simulink model "ES005A_TmplMonr"  (R2013b)
settings: Solver=ode45  StartTime=0.0  StopTime=2  RelTol=1e-3
values from neighbouring files (symbols this model uses):
  ELECGLBPRM_STRTUPSTTMPLMONININTESTSTRT_CNT_U08 = DataDict.Constant    [ES005A_TmplMonr_DataDict.m]
  IninFlt = DataDict.NTC    [ES005A_TmplMonr_DataDict.m]
  RtFlt = DataDict.NTC    [ES005A_TmplMonr_DataDict.m]
  SpiConf_SpiChannel_TmplMonrCh1 = DataDict.Constant    [ES005A_TmplMonr_DataDict.m]
  SpiConf_SpiChannel_TmplMonrCh2 = DataDict.Constant    [ES005A_TmplMonr_DataDict.m]
  SpiConf_SpiChannel_TmplMonrCh3 = DataDict.Constant    [ES005A_TmplMonr_DataDict.m]
  SpiConf_SpiSequence_TmplMonrSeq1 = DataDict.Constant    [ES005A_TmplMonr_DataDict.m]
  SpiConf_SpiSequence_TmplMonrSeq2 = DataDict.Constant    [ES005A_TmplMonr_DataDict.m]
  SpiConf_SpiSequence_TmplMonrSeq3 = DataDict.Constant    [ES005A_TmplMonr_DataDict.m]
  STD_HIGH = DataDict.Constant    [ES005A_TmplMonr_DataDict.m]
  STD_LOW = DataDict.Constant    [ES005A_TmplMonr_DataDict.m]
  TMPLMONRCFGREG1READVAL_CNT_U16 = DataDict.Constant    [ES005A_TmplMonr_DataDict.m]
  TMPLMONRCFGREG1WRVAL_CNT_U16 = DataDict.Constant    [ES005A_TmplMonr_DataDict.m]
  TMPLMONRSTSREG2READVAL_CNT_U16 = DataDict.Constant    [ES005A_TmplMonr_DataDict.m]
  TMPLMONRWDGMODKEYWORD1_CNT_U16 = DataDict.Constant    [ES005A_TmplMonr_DataDict.m]
  TMPLMONRWDGMODKEYWORD2_CNT_U16 = DataDict.Constant    [ES005A_TmplMonr_DataDict.m]
  TMPLMONRWDGMODKEYWORD3_CNT_U16 = DataDict.Constant    [ES005A_TmplMonr_DataDict.m]
undefined symbols (not defined in the file or in its folder): TrigReg1
libraries: simulink x12
(part 2 of 4)

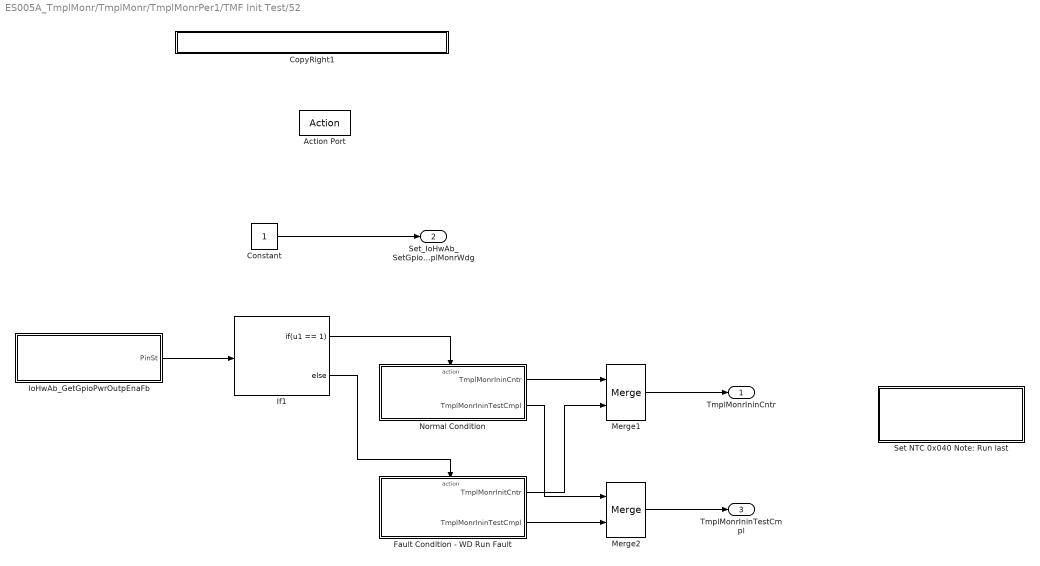
== system ES005A_TmplMonr/TmplMonr/TmplMonrPer1/TMF Init Test/52 ==
  Action Port : ActionPort  ActionType=case
  Constant : Constant  OutDataTypeStr=boolean
  CopyRight1 : Subsystem  Description=|  mask(Copyright Information){none=on}
      | Copyright info block.                                               
      |                                                                     
      | Place copyright information at the top of every subsystem in design.
      mask prompts: none "No parameters"
      mask help: Place copyright information at the top of every subsystem in design.
      mask Display:
      | NxtrConf = 'Nexteer Confidential';
      | 
      | sys = bdroot; %handle for the current model ("system")
      | first = get_param(sys,'Created');
      | first = first(end-3:end);  %year is last four digits
      | 
      | last = get_param(sys,'LastModifiedDate');
      | if isempty(last)
      |     last = datestr(now,'yyyy');
      | else
      |     last = last(end-3:end);
      | end
      | 
      | if strcmp(first,last)
      |     fprintf('%s -- Copyright %s Nexteer',NxtrConf,first)
      | else
      |     fprintf('%s -- %s%s- %s Nexteer',NxtrConf,char(169),first,last)
      | end
  Fault Condition - WD Run Fault : Subsystem  RequirementInfo={} %GIDa_b93698f8_2763_40bb_9d1b_225acd7973d3
  If1 : If  IfExpression=u1 == 1
  IoHwAb_GetGpioPwrOutpEnaFb : Subsystem
  Merge1 : Merge
  Merge2 : Merge
  Normal Condition : Subsystem  RequirementInfo={'linktype_rmi_doors' '0000c46a (/ESG Group/FDD Module Requirements/EA4 Specific/ES005A_TmplMonr)' '#ES005A_164' 'true' 'REQ: ES005A_164' '' } %GIDa_785a744b_ba8b_461e_b98b_5c61c0bc0772
  Set NTC 0x040 Note: Run last : Subsystem  RequirementInfo="{'linktype_rmi_doors' '0000c46a (/ESG Group/FDD Module Requirements/EA4 Specific/ES005A_TmplMonr)' '#ES005A_183' 'true' 'REQ:  ES005A_183' '' } %GIDa_d81dec6a_41a1_4ea0_a985_1fcdbb0d2b96"
  TmplMonrIninCntr : Outport
  Set_IoHwAb_SetGpioTmplMonrWdg : Outport  Port=2
  TmplMonrIninTestCmpl : Outport  Port=3
  wires:
  If1/1 -> Normal Condition/Action
  If1/2 -> Fault Condition - WD Run Fault/Action
  IoHwAb_GetGpioPwrOutpEnaFb/1(PinSt) -> If1/1
  Normal Condition/1(TmplMonrIninCntr) -> Merge1/1
  Fault Condition - WD Run Fault/1(TmplMonrInitCntr) -> Merge1/2
  Constant/1 -> Set_IoHwAb_SetGpioTmplMonrWdg/1
  Merge1/1 -> TmplMonrIninCntr/1
  Merge2/1 -> TmplMonrIninTestCmpl/1
  Normal Condition/2(TmplMonrIninTestCmpl) -> Merge2/1
  Fault Condition - WD Run Fault/2(TmplMonrIninTestCmpl) -> Merge2/2

== system ES005A_TmplMonr/TmplMonr/TmplMonrPer1/TMF Init Test/9-10, 14-16 ==
  Action Port : ActionPort  ActionType=case
  Constant : Constant  Value=0  OutDataTypeStr=boolean
  Constant2 : Constant  OutDataTypeStr=uint8
  Constant3 : Constant  Value=STD_HIGH  OutDataTypeStr=boolean
  CopyRight1 : Subsystem  Description=|  mask(Copyright Information){none=on}
      | Copyright info block.                                               
      |                                                                     
      | Place copyright information at the top of every subsystem in design.
      mask prompts: none "No parameters"
      mask help: Place copyright information at the top of every subsystem in design.
      mask Display:
      | NxtrConf = 'Nexteer Confidential';
      | 
      | sys = bdroot; %handle for the current model ("system")
      | first = get_param(sys,'Created');
      | first = first(end-3:end);  %year is last four digits
      | 
      | last = get_param(sys,'LastModifiedDate');
      | if isempty(last)
      |     last = datestr(now,'yyyy');
      | else
      |     last = last(end-3:end);
      | end
      | 
      | if strcmp(first,last)
      |     fprintf('%s -- Copyright %s Nexteer',NxtrConf,first)
      | else
      |     fprintf('%s -- %s%s- %s Nexteer',NxtrConf,char(169),first,last)
      | end
  Data Store Read1 : DataStoreRead  DataStoreName=TmplMonrIninCntr
  If2 : If  RequirementInfo={'linktype_rmi_doors' '0000c46a (/ESG Group/FDD Module Requirements/EA4 Specific/ES005A_TmplMonr)' '#ES005A_163' 'true' 'REQ: ES005A_163' '' ; 'linktype_rmi_doors' '0000c46a (/ESG Group/FDD Module Requirements/EA4 Specific/ES005A_TmplMonr)' '#ES005A_172' 'true' 'REQ: ES005A_172' '' } %GIDa_befe16eb_941f_4fe1_a71f_516baf802abf  IfExpression=u1 < 16  ShowElse=off
  IoHwAb_GetGpioPwrOutpEnaFb1 : Subsystem
  TmplMonrIninCntr : Outport
  Set_IoHwAb_SetGpioTmplMonrWdg : Outport  Port=2
  nErr : Outport  Port=3
  wires:
  Constant2/1 -> TmplMonrIninCntr/1
  Constant/1 -> Set_IoHwAb_SetGpioTmplMonrWdg/1
  Constant3/1 -> nErr/1
  If2/1 -> IoHwAb_GetGpioPwrOutpEnaFb1/Action
  Data Store Read1/1 -> If2/1

== system ES005A_TmplMonr/TmplMonr/TmplMonrPer1/TMF Init Test/CopyRight1 ==

== system ES005A_TmplMonr/TmplMonr/TmplMonrPer1/TMF Init Test/Default ==
  note: DO NOTHING
  Action Port : ActionPort  ActionType=default
  CopyRight1 : Subsystem  Description=|  mask(Copyright Information){none=on}
      | Copyright info block.                                               
      |                                                                     
      | Place copyright information at the top of every subsystem in design.
      mask prompts: none "No parameters"
      mask help: Place copyright information at the top of every subsystem in design.
      mask Display:
      | NxtrConf = 'Nexteer Confidential';
      | 
      | sys = bdroot; %handle for the current model ("system")
      | first = get_param(sys,'Created');
      | first = first(end-3:end);  %year is last four digits
      | 
      | last = get_param(sys,'LastModifiedDate');
      | if isempty(last)
      |     last = datestr(now,'yyyy');
      | else
      |     last = last(end-3:end);
      | end
      | 
      | if strcmp(first,last)
      |     fprintf('%s -- Copyright %s Nexteer',NxtrConf,first)
      | else
      |     fprintf('%s -- %s%s- %s Nexteer',NxtrConf,char(169),first,last)
      | end

== system ES005A_TmplMonr/TmplMonr/TmplMonrPer1/TMF Init Test/IoHwAb_SetGpioTmplMonrWdg ==
  Trigger : TriggerPort  PortDimensions=1
  Constant1 : Constant  OutDataTypeStr=boolean
  CopyRight1 : Subsystem  Description=|  mask(Copyright Information){none=on}
      | Copyright info block.                                               
      |                                                                     
      | Place copyright information at the top of every subsystem in design.
      mask prompts: none "No parameters"
      mask help: Place copyright information at the top of every subsystem in design.
      mask Display:
      | NxtrConf = 'Nexteer Confidential';
      | 
      | sys = bdroot; %handle for the current model ("system")
      | first = get_param(sys,'Created');
      | first = first(end-3:end);  %year is last four digits
      | 
      | last = get_param(sys,'LastModifiedDate');
      | if isempty(last)
      |     last = datestr(now,'yyyy');
      | else
      |     last = last(end-3:end);
      | end
      | 
      | if strcmp(first,last)
      |     fprintf('%s -- Copyright %s Nexteer',NxtrConf,first)
      | else
      |     fprintf('%s -- %s%s- %s Nexteer',NxtrConf,char(169),first,last)
      | end
  IoHwAb_SetGpioTmplMonrWdg : Subsystem
  wires:
  Constant1/1 -> IoHwAb_SetGpioTmplMonrWdg/1(PinSt)

== system ES005A_TmplMonr/TmplMonr/TmplMonrPer1/TMF Init Test/nError Signal Control ==
  NerrSt : Inport  RequirementInfo={} %GIDa_e0111a0c_ce8f_4caa_a82b_fb1ad2110f0d
  CopyRight1 : Subsystem  Description=|  mask(Copyright Information){none=on}
      | Copyright info block.                                               
      |                                                                     
      | Place copyright information at the top of every subsystem in design.
      mask prompts: none "No parameters"
      mask help: Place copyright information at the top of every subsystem in design.
      mask Display:
      | NxtrConf = 'Nexteer Confidential';
      | 
      | sys = bdroot; %handle for the current model ("system")
      | first = get_param(sys,'Created');
      | first = first(end-3:end);  %year is last four digits
      | 
      | last = get_param(sys,'LastModifiedDate');
      | if isempty(last)
      |     last = datestr(now,'yyyy');
      | else
      |     last = last(end-3:end);
      | end
      | 
      | if strcmp(first,last)
      |     fprintf('%s -- Copyright %s Nexteer',NxtrConf,first)
      | else
      |     fprintf('%s -- %s%s- %s Nexteer',NxtrConf,char(169),first,last)
      | end
  "CtrlErrOut " : Subsystem
  NtcNr2 : simulink/Sources/Enumerated Constant  OutDataTypeStr=Enum: TrigReg1  Value=TrigReg1.TRIGREG_MSTANDCHKR  SampleTime=inf
  wires:
  NerrSt/1 -> "CtrlErrOut "/1(PinSt_ArgIn)
  NtcNr2/1 -> "CtrlErrOut "/2(TrigReg_ArgIn)

== system ES005A_TmplMonr/TmplMonr/TmplMonrPer1/TMF Run/CopyRight1 ==

== system ES005A_TmplMonr/TmplMonr/TmplMonrPer1/TMF Run/Fault Condition - WD Run Fault ==
  Action Port : ActionPort  ActionType=else
  CopyRight1 : Subsystem  Description=|  mask(Copyright Information){none=on}
      | Copyright info block.                                               
      |                                                                     
      | Place copyright information at the top of every subsystem in design.
      mask prompts: none "No parameters"
      mask help: Place copyright information at the top of every subsystem in design.
      mask Display:
      | NxtrConf = 'Nexteer Confidential';
      | 
      | sys = bdroot; %handle for the current model ("system")
      | first = get_param(sys,'Created');
      | first = first(end-3:end);  %year is last four digits
      | 
      | last = get_param(sys,'LastModifiedDate');
      | if isempty(last)
      |     last = datestr(now,'yyyy');
      | else
      |     last = last(end-3:end);
      | end
      | 
      | if strcmp(first,last)
      |     fprintf('%s -- Copyright %s Nexteer',NxtrConf,first)
      | else
      |     fprintf('%s -- %s%s- %s Nexteer',NxtrConf,char(169),first,last)
      | end
  Data Store Read1 : DataStoreRead  DataStoreName=TmplMonrSpiReadWrOrderFlg2
  If : If  IfExpression=u1 == 0
  "TmplMonrSpiReadWrOrderFlg2 = 0 (Read Cmd) " : Subsystem
  TmplMonrSpiReadWrOrderFlg2 = 1 (Read Buffer) : Subsystem
  wires:
  If/1 -> "TmplMonrSpiReadWrOrderFlg2 = 0 (Read Cmd) "/Action
  If/2 -> TmplMonrSpiReadWrOrderFlg2 = 1 (Read Buffer)/Action
  Data Store Read1/1 -> If/1

== system ES005A_TmplMonr/TmplMonr/TmplMonrPer1/TMF Run/IoHwAb_GetGpioPwrOutpEnaFb ==
  CopyRight1 : Subsystem  Description=|  mask(Copyright Information){none=on}
      | Copyright info block.                                               
      |                                                                     
      | Place copyright information at the top of every subsystem in design.
      mask prompts: none "No parameters"
      mask help: Place copyright information at the top of every subsystem in design.
      mask Display:
      | NxtrConf = 'Nexteer Confidential';
      | 
      | sys = bdroot; %handle for the current model ("system")
      | first = get_param(sys,'Created');
      | first = first(end-3:end);  %year is last four digits
      | 
      | last = get_param(sys,'LastModifiedDate');
      | if isempty(last)
      |     last = datestr(now,'yyyy');
      | else
      |     last = last(end-3:end);
      | end
      | 
      | if strcmp(first,last)
      |     fprintf('%s -- Copyright %s Nexteer',NxtrConf,first)
      | else
      |     fprintf('%s -- %s%s- %s Nexteer',NxtrConf,char(169),first,last)
      | end
  Ground : Ground
  PinSt : Outport
  wires:
  Ground/1 -> PinSt/1

== system ES005A_TmplMonr/TmplMonr/TmplMonrPer1/TMF Run/IoHwAb_SetGpioTmplMonrWdg1 ==
  PinSt : Inport
  CopyRight1 : Subsystem  Description=|  mask(Copyright Information){none=on}
      | Copyright info block.                                               
      |                                                                     
      | Place copyright information at the top of every subsystem in design.
      mask prompts: none "No parameters"
      mask help: Place copyright information at the top of every subsystem in design.
      mask Display:
      | NxtrConf = 'Nexteer Confidential';
      | 
      | sys = bdroot; %handle for the current model ("system")
      | first = get_param(sys,'Created');
      | first = first(end-3:end);  %year is last four digits
      | 
      | last = get_param(sys,'LastModifiedDate');
      | if isempty(last)
      |     last = datestr(now,'yyyy');
      | else
      |     last = last(end-3:end);
      | end
      | 
      | if strcmp(first,last)
      |     fprintf('%s -- Copyright %s Nexteer',NxtrConf,first)
      | else
      |     fprintf('%s -- %s%s- %s Nexteer',NxtrConf,char(169),first,last)
      | end
  Terminator : Terminator
  wires:
  PinSt/1 -> Terminator/1

== system ES005A_TmplMonr/TmplMonr/TmplMonrPer1/TMF Run/Normal Condition ==
  Action Port : ActionPort  ActionType=then
  Constant1 : Constant  Value=0  OutDataTypeStr=boolean
  CopyRight1 : Subsystem  Description=|  mask(Copyright Information){none=on}
      | Copyright info block.                                               
      |                                                                     
      | Place copyright information at the top of every subsystem in design.
      mask prompts: none "No parameters"
      mask help: Place copyright information at the top of every subsystem in design.
      mask Display:
      | NxtrConf = 'Nexteer Confidential';
      | 
      | sys = bdroot; %handle for the current model ("system")
      | first = get_param(sys,'Created');
      | first = first(end-3:end);  %year is last four digits
      | 
      | last = get_param(sys,'LastModifiedDate');
      | if isempty(last)
      |     last = datestr(now,'yyyy');
      | else
      |     last = last(end-3:end);
      | end
      | 
      | if strcmp(first,last)
      |     fprintf('%s -- Copyright %s Nexteer',NxtrConf,first)
      | else
      |     fprintf('%s -- %s%s- %s Nexteer',NxtrConf,char(169),first,last)
      | end
  Data Store Write : DataStoreWrite  DataStoreName=TmplMonrSpiReadWrOrderFlg2
  NtcNr1 : Constant  Value=RtFlt
  NtcStInfo : Constant  Value=0  OutDataTypeStr=uint8
  NtcSts : Constant  Value=0  OutDataTypeStr=uint8
  SetNtcSts : Subsystem
  non debounce : Constant  Value=0  OutDataTypeStr=uint16
  wires:
  NtcNr1/1 -> SetNtcSts/1(NtcNr)
  non debounce/1 -> SetNtcSts/4(DebStep)
  NtcSts/1 -> SetNtcSts/3(NtcSts)
  NtcStInfo/1 -> SetNtcSts/2(NtcStInfo)
  Constant1/1 -> Data Store Write/1

== system ES005A_TmplMonr/TmplMonr/TmplMonrPer1/TMF Init Test/0-8/CopyRight1 ==

== system ES005A_TmplMonr/TmplMonr/TmplMonrPer1/TMF Init Test/11/CopyRight1 ==

== system ES005A_TmplMonr/TmplMonr/TmplMonrPer1/TMF Init Test/12/CopyRight1 ==

== system ES005A_TmplMonr/TmplMonr/TmplMonrPer1/TMF Init Test/12/Fault Condition - AND Gate ==
  note: NTCNR_0X040
      | Parameters:
      |     1 = 0000 0001 = Bit 0 = Fault Occured Between TmplMonrInitCntr =  9 ~ 10
      |     2 = 0000 0010 = Bit 1 = Fault Occured Between TmplMonrInitCntr = 12 (AND Gate Fault)
      |     4 = 0000 0100 = Bit 2 = Fault Occured Between TmplMonrInitCntr = 14 ~ 15
      |     8 = 0000 1000 = Bit 3 = Fault Occured at TmplMonrInitCntr            = 17  (POE Fault)
      |   16 = 0001 0000 = Bit 4 = Fault Occured at TmplMonrInitCntr            = 18 (WD_STATE Fault)
      |   32 = 0010 0000 = Bit 5 = Fault Occured at TmplMonrInitCntr            = 20 (Edge/Valid Write Fault)
      |   64 = 0100 0000 = Bit 6 = Fault Occured at TmplMonrInitCntr            = 52 (POE + Non-WD Fault)
      | 128 = 1000 0000 = Bit 7 = Fault Occured at TmplMonrInitCntr            = 52 (POE + WD Fault)
  Action Port : ActionPort  ActionType=then
  Bitwise Operator2 : simulink/Logic and Bit Operations/Bitwise Operator  logicop=OR  UseBitMask=off  NumInputPorts=2  BitMask=bin2dec('00001111')  BitMaskRealWorld=Stored Integer
  CopyRight1 : Subsystem  Description=|  mask(Copyright Information){none=on}
      | Copyright info block.                                               
      |                                                                     
      | Place copyright information at the top of every subsystem in design.
      mask prompts: none "No parameters"
      mask help: Place copyright information at the top of every subsystem in design.
      mask Display:
      | NxtrConf = 'Nexteer Confidential';
      | 
      | sys = bdroot; %handle for the current model ("system")
      | first = get_param(sys,'Created');
      | first = first(end-3:end);  %year is last four digits
      | 
      | last = get_param(sys,'LastModifiedDate');
      | if isempty(last)
      |     last = datestr(now,'yyyy');
      | else
      |     last = last(end-3:end);
      | end
      | 
      | if strcmp(first,last)
      |     fprintf('%s -- Copyright %s Nexteer',NxtrConf,first)
      | else
      |     fprintf('%s -- %s%s- %s Nexteer',NxtrConf,char(169),first,last)
      | end
  Data Store Read3 : DataStoreRead  DataStoreName=TmplMonrNtc40PrmByte  DataStoreElements=TmplMonrNtc40PrmByte
  Data Store Write1 : DataStoreWrite  DataStoreName=TmplMonrNtc40PrmByte
  NtcStInfo : Constant  Value=2  OutDataTypeStr=uint8
  wires:
  Bitwise Operator2/1 -> Data Store Write1/1
  Data Store Read3/1 -> Bitwise Operator2/1
  NtcStInfo/1 -> Bitwise Operator2/2

== system ES005A_TmplMonr/TmplMonr/TmplMonrPer1/TMF Init Test/12/IoHwAb_GetGpioPwrOutpEnaFb ==
  CopyRight1 : Subsystem  Description=|  mask(Copyright Information){none=on}
      | Copyright info block.                                               
      |                                                                     
      | Place copyright information at the top of every subsystem in design.
      mask prompts: none "No parameters"
      mask help: Place copyright information at the top of every subsystem in design.
      mask Display:
      | NxtrConf = 'Nexteer Confidential';
      | 
      | sys = bdroot; %handle for the current model ("system")
      | first = get_param(sys,'Created');
      | first = first(end-3:end);  %year is last four digits
      | 
      | last = get_param(sys,'LastModifiedDate');
      | if isempty(last)
      |     last = datestr(now,'yyyy');
      | else
      |     last = last(end-3:end);
      | end
      | 
      | if strcmp(first,last)
      |     fprintf('%s -- Copyright %s Nexteer',NxtrConf,first)
      | else
      |     fprintf('%s -- %s%s- %s Nexteer',NxtrConf,char(169),first,last)
      | end
  Ground : Ground
  PinSt : Outport
  wires:
  Ground/1 -> PinSt/1

== system ES005A_TmplMonr/TmplMonr/TmplMonrPer1/TMF Init Test/13/CopyRight1 ==

== system ES005A_TmplMonr/TmplMonr/TmplMonrPer1/TMF Init Test/17/Call_Spi_AsyncTransmit ==
  Sequence : Inport
  CopyRight1 : Subsystem  Description=|  mask(Copyright Information){none=on}
      | Copyright info block.                                               
      |                                                                     
      | Place copyright information at the top of every subsystem in design.
      mask prompts: none "No parameters"
      mask help: Place copyright information at the top of every subsystem in design.
      mask Display:
      | NxtrConf = 'Nexteer Confidential';
      | 
      | sys = bdroot; %handle for the current model ("system")
      | first = get_param(sys,'Created');
      | first = first(end-3:end);  %year is last four digits
      | 
      | last = get_param(sys,'LastModifiedDate');
      | if isempty(last)
      |     last = datestr(now,'yyyy');
      | else
      |     last = last(end-3:end);
      | end
      | 
      | if strcmp(first,last)
      |     fprintf('%s -- Copyright %s Nexteer',NxtrConf,first)
      | else
      |     fprintf('%s -- %s%s- %s Nexteer',NxtrConf,char(169),first,last)
      | end
  Terminator : Terminator
  wires:
  Sequence/1 -> Terminator/1

== system ES005A_TmplMonr/TmplMonr/TmplMonrPer1/TMF Init Test/17/CopyRight1 ==

== system ES005A_TmplMonr/TmplMonr/TmplMonrPer1/TMF Init Test/17/Fault Condition - WD ==
  note: NTCNR_0X040
      | Parameters:
      |     1 = 0000 0001 = Bit 0 = Fault Occured Between TmplMonrInitCntr =  9 ~ 10
      |     2 = 0000 0010 = Bit 1 = Fault Occured Between TmplMonrInitCntr = 12 (AND Gate Fault)
      |     4 = 0000 0100 = Bit 2 = Fault Occured Between TmplMonrInitCntr = 14 ~ 15
      |     8 = 0000 1000 = Bit 3 = Fault Occured at TmplMonrInitCntr            = 17  (POE Fault)
      |   16 = 0001 0000 = Bit 4 = Fault Occured at TmplMonrInitCntr            = 18 (WD_STATE Fault)
      |   32 = 0010 0000 = Bit 5 = Fault Occured at TmplMonrInitCntr            = 20 (Edge/Valid Write Fault)
      |   64 = 0100 0000 = Bit 6 = Fault Occured at TmplMonrInitCntr            = 52 (POE + Non-WD Fault)
      | 128 = 1000 0000 = Bit 7 = Fault Occured at TmplMonrInitCntr            = 52 (POE + WD Fault)
  Action Port : ActionPort  ActionType=then
  Bitwise Operator2 : simulink/Logic and Bit Operations/Bitwise Operator  logicop=OR  UseBitMask=off  NumInputPorts=2  BitMask=bin2dec('00001111')  BitMaskRealWorld=Stored Integer
  CopyRight1 : Subsystem  Description=|  mask(Copyright Information){none=on}
      | Copyright info block.                                               
      |                                                                     
      | Place copyright information at the top of every subsystem in design.
      mask prompts: none "No parameters"
      mask help: Place copyright information at the top of every subsystem in design.
      mask Display:
      | NxtrConf = 'Nexteer Confidential';
      | 
      | sys = bdroot; %handle for the current model ("system")
      | first = get_param(sys,'Created');
      | first = first(end-3:end);  %year is last four digits
      | 
      | last = get_param(sys,'LastModifiedDate');
      | if isempty(last)
      |     last = datestr(now,'yyyy');
      | else
      |     last = last(end-3:end);
      | end
      | 
      | if strcmp(first,last)
      |     fprintf('%s -- Copyright %s Nexteer',NxtrConf,first)
      | else
      |     fprintf('%s -- %s%s- %s Nexteer',NxtrConf,char(169),first,last)
      | end
  Data Store Read3 : DataStoreRead  DataStoreName=TmplMonrNtc40PrmByte  DataStoreElements=TmplMonrNtc40PrmByte
  Data Store Write1 : DataStoreWrite  DataStoreName=TmplMonrNtc40PrmByte
  NtcStInfo : Constant  Value=8  OutDataTypeStr=uint8
  wires:
  Bitwise Operator2/1 -> Data Store Write1/1
  Data Store Read3/1 -> Bitwise Operator2/1
  NtcStInfo/1 -> Bitwise Operator2/2

== system ES005A_TmplMonr/TmplMonr/TmplMonrPer1/TMF Init Test/17/IoHwAb_GetGpioPwrOutpEnaFb ==
  CopyRight1 : Subsystem  Description=|  mask(Copyright Information){none=on}
      | Copyright info block.                                               
      |                                                                     
      | Place copyright information at the top of every subsystem in design.
      mask prompts: none "No parameters"
      mask help: Place copyright information at the top of every subsystem in design.
      mask Display:
      | NxtrConf = 'Nexteer Confidential';
      | 
      | sys = bdroot; %handle for the current model ("system")
      | first = get_param(sys,'Created');
      | first = first(end-3:end);  %year is last four digits
      | 
      | last = get_param(sys,'LastModifiedDate');
      | if isempty(last)
      |     last = datestr(now,'yyyy');
      | else
      |     last = last(end-3:end);
      | end
      | 
      | if strcmp(first,last)
      |     fprintf('%s -- Copyright %s Nexteer',NxtrConf,first)
      | else
      |     fprintf('%s -- %s%s- %s Nexteer',NxtrConf,char(169),first,last)
      | end
  Ground : Ground
  PinSt : Outport
  wires:
  Ground/1 -> PinSt/1

== system ES005A_TmplMonr/TmplMonr/TmplMonrPer1/TMF Init Test/17/Spi_WriteIB ==
  Channel : Inport
  DataBufferPtr : Inport  Port=2
  CopyRight1 : Subsystem  Description=|  mask(Copyright Information){none=on}
      | Copyright info block.                                               
      |                                                                     
      | Place copyright information at the top of every subsystem in design.
      mask prompts: none "No parameters"
      mask help: Place copyright information at the top of every subsystem in design.
      mask Display:
      | NxtrConf = 'Nexteer Confidential';
      | 
      | sys = bdroot; %handle for the current model ("system")
      | first = get_param(sys,'Created');
      | first = first(end-3:end);  %year is last four digits
      | 
      | last = get_param(sys,'LastModifiedDate');
      | if isempty(last)
      |     last = datestr(now,'yyyy');
      | else
      |     last = last(end-3:end);
      | end
      | 
      | if strcmp(first,last)
      |     fprintf('%s -- Copyright %s Nexteer',NxtrConf,first)
      | else
      |     fprintf('%s -- %s%s- %s Nexteer',NxtrConf,char(169),first,last)
      | end
  Terminator : Terminator
  Terminator1 : Terminator
  wires:
  Channel/1 -> Terminator/1
  DataBufferPtr/1 -> Terminator1/1

== system ES005A_TmplMonr/TmplMonr/TmplMonrPer1/TMF Init Test/18/CopyRight1 ==

== system ES005A_TmplMonr/TmplMonr/TmplMonrPer1/TMF Init Test/18/Spi_ReadIB ==
  note: 00101100
  note: Read Buffer - Simulation Purpose Only
  Channel : Inport
  Constant3 : Constant  Value=44  OutDataTypeStr=uint16
  CopyRight1 : Subsystem  Description=|  mask(Copyright Information){none=on}
      | Copyright info block.                                               
      |                                                                     
      | Place copyright information at the top of every subsystem in design.
      mask prompts: none "No parameters"
      mask help: Place copyright information at the top of every subsystem in design.
      mask Display:
      | NxtrConf = 'Nexteer Confidential';
      | 
      | sys = bdroot; %handle for the current model ("system")
      | first = get_param(sys,'Created');
      | first = first(end-3:end);  %year is last four digits
      | 
      | last = get_param(sys,'LastModifiedDate');
      | if isempty(last)
      |     last = datestr(now,'yyyy');
      | else
      |     last = last(end-3:end);
      | end
      | 
      | if strcmp(first,last)
      |     fprintf('%s -- Copyright %s Nexteer',NxtrConf,first)
      | else
      |     fprintf('%s -- %s%s- %s Nexteer',NxtrConf,char(169),first,last)
      | end
  Terminator : Terminator
  Rx : Outport
  wires:
  Constant3/1 -> Rx/1
  Channel/1 -> Terminator/1

== system ES005A_TmplMonr/TmplMonr/TmplMonrPer1/TMF Init Test/18/WD_STATE = 0 ~ 2, 7 ==
  note: NTCNR_0X040
      | Parameters:
      |     1 = 0000 0001 = Bit 0 = Fault Occured Between TmplMonrInitCntr =  9 ~ 10
      |     2 = 0000 0010 = Bit 1 = Fault Occured Between TmplMonrInitCntr = 12 (AND Gate Fault)
      |     4 = 0000 0100 = Bit 2 = Fault Occured Between TmplMonrInitCntr = 14 ~ 15
      |     8 = 0000 1000 = Bit 3 = Fault Occured at TmplMonrInitCntr            = 17  (POE Fault)
      |   16 = 0001 0000 = Bit 4 = Fault Occured at TmplMonrInitCntr            = 18 (WD_STATE Fault)
      |   32 = 0010 0000 = Bit 5 = Fault Occured at TmplMonrInitCntr            = 20 (Edge/Valid Write Fault)
      |   64 = 0100 0000 = Bit 6 = Fault Occured at TmplMonrInitCntr            = 52 (POE + Non-WD Fault)
      | 128 = 1000 0000 = Bit 7 = Fault Occured at TmplMonrInitCntr            = 52 (POE + WD Fault)
  Action Port : ActionPort  ActionType=else
  Constant2 : Constant  Value=0  OutDataTypeStr=uint8
  CopyRight1 : Subsystem  Description=|  mask(Copyright Information){none=on}
      | Copyright info block.                                               
      |                                                                     
      | Place copyright information at the top of every subsystem in design.
      mask prompts: none "No parameters"
      mask help: Place copyright information at the top of every subsystem in design.
      mask Display:
      | NxtrConf = 'Nexteer Confidential';
      | 
      | sys = bdroot; %handle for the current model ("system")
      | first = get_param(sys,'Created');
      | first = first(end-3:end);  %year is last four digits
      | 
      | last = get_param(sys,'LastModifiedDate');
      | if isempty(last)
      |     last = datestr(now,'yyyy');
      | else
      |     last = last(end-3:end);
      | end
      | 
      | if strcmp(first,last)
      |     fprintf('%s -- Copyright %s Nexteer',NxtrConf,first)
      | else
      |     fprintf('%s -- %s%s- %s Nexteer',NxtrConf,char(169),first,last)
      | end
  Data Store Read1 : DataStoreRead  DataStoreName=TmplMonrWdgRstrtCnt
  If : If  IfExpression=u1 <= 1
  Jump to Stage 52 : Subsystem
  WD RESTART - Two Re-try : Subsystem
  TmplMonrIninCntr : Outport
  wires:
  If/1 -> WD RESTART - Two Re-try/Action
  If/2 -> Jump to Stage 52/Action
  Data Store Read1/1 -> If/1
  Constant2/1 -> TmplMonrIninCntr/1

== system ES005A_TmplMonr/TmplMonr/TmplMonrPer1/TMF Init Test/18/WD_STATE = 3 ~ 6 ==
  note: Write: Edge/Valid - 10011000001011
  Action Port : ActionPort  ActionType=then
  Call_Spi_AsyncTransmit : Subsystem
  Constant1 : Constant  Value=SpiConf_SpiSequence_TmplMonrSeq2  OutDataTypeStr=boolean
  Constant2 : Constant  OutDataTypeStr=uint8
  Constant4 : Constant  Value=SpiConf_SpiChannel_TmplMonrCh2  OutDataTypeStr=boolean
  Constant5 : Constant  Value=TMPLMONRCFGREG1WRVAL_CNT_U16  OutDataTypeStr=uint16
  CopyRight1 : Subsystem  Description=|  mask(Copyright Information){none=on}
      | Copyright info block.                                               
      |                                                                     
      | Place copyright information at the top of every subsystem in design.
      mask prompts: none "No parameters"
      mask help: Place copyright information at the top of every subsystem in design.
      mask Display:
      | NxtrConf = 'Nexteer Confidential';
      | 
      | sys = bdroot; %handle for the current model ("system")
      | first = get_param(sys,'Created');
      | first = first(end-3:end);  %year is last four digits
      | 
      | last = get_param(sys,'LastModifiedDate');
      | if isempty(last)
      |     last = datestr(now,'yyyy');
      | else
      |     last = last(end-3:end);
      | end
      | 
      | if strcmp(first,last)
      |     fprintf('%s -- Copyright %s Nexteer',NxtrConf,first)
      | else
      |     fprintf('%s -- %s%s- %s Nexteer',NxtrConf,char(169),first,last)
      | end
  Spi_WriteIB : Subsystem
  TmplMonrIninCntr : Outport
  wires:
  Constant1/1 -> Call_Spi_AsyncTransmit/1(Sequence)
  Constant4/1 -> Spi_WriteIB/1(Channel)
  Constant5/1 -> Spi_WriteIB/2(DataBufferPtr)
  Constant2/1 -> TmplMonrIninCntr/1

== system ES005A_TmplMonr/TmplMonr/TmplMonrPer1/TMF Init Test/19/Call_Spi_AsyncTransmit ==
  Sequence : Inport
  CopyRight1 : Subsystem  Description=|  mask(Copyright Information){none=on}
      | Copyright info block.                                               
      |                                                                     
      | Place copyright information at the top of every subsystem in design.
      mask prompts: none "No parameters"
      mask help: Place copyright information at the top of every subsystem in design.
      mask Display:
      | NxtrConf = 'Nexteer Confidential';
      | 
      | sys = bdroot; %handle for the current model ("system")
      | first = get_param(sys,'Created');
      | first = first(end-3:end);  %year is last four digits
      | 
      | last = get_param(sys,'LastModifiedDate');
      | if isempty(last)
      |     last = datestr(now,'yyyy');
      | else
      |     last = last(end-3:end);
      | end
      | 
      | if strcmp(first,last)
      |     fprintf('%s -- Copyright %s Nexteer',NxtrConf,first)
      | else
      |     fprintf('%s -- %s%s- %s Nexteer',NxtrConf,char(169),first,last)
      | end
  Terminator : Terminator
  wires:
  Sequence/1 -> Terminator/1

== system ES005A_TmplMonr/TmplMonr/TmplMonrPer1/TMF Init Test/19/CopyRight1 ==

== system ES005A_TmplMonr/TmplMonr/TmplMonrPer1/TMF Init Test/19/Spi_WriteIB ==
  Channel : Inport
  DataBufferPtr : Inport  Port=2
  CopyRight1 : Subsystem  Description=|  mask(Copyright Information){none=on}
      | Copyright info block.                                               
      |                                                                     
      | Place copyright information at the top of every subsystem in design.
      mask prompts: none "No parameters"
      mask help: Place copyright information at the top of every subsystem in design.
      mask Display:
      | NxtrConf = 'Nexteer Confidential';
      | 
      | sys = bdroot; %handle for the current model ("system")
      | first = get_param(sys,'Created');
      | first = first(end-3:end);  %year is last four digits
      | 
      | last = get_param(sys,'LastModifiedDate');
      | if isempty(last)
      |     last = datestr(now,'yyyy');
      | else
      |     last = last(end-3:end);
      | end
      | 
      | if strcmp(first,last)
      |     fprintf('%s -- Copyright %s Nexteer',NxtrConf,first)
      | else
      |     fprintf('%s -- %s%s- %s Nexteer',NxtrConf,char(169),first,last)
      | end
  Terminator : Terminator
  Terminator1 : Terminator
  wires:
  Channel/1 -> Terminator/1
  DataBufferPtr/1 -> Terminator1/1

== system ES005A_TmplMonr/TmplMonr/TmplMonrPer1/TMF Init Test/20/CopyRight1 ==

== system ES005A_TmplMonr/TmplMonr/TmplMonrPer1/TMF Init Test/20/Edge//Valid Cnts are NOT Correct ==
  note: NTCNR_0X040
      | Parameters:
      |     1 = 0000 0001 = Bit 0 = Fault Occured Between TmplMonrInitCntr =  9 ~ 10
      |     2 = 0000 0010 = Bit 1 = Fault Occured Between TmplMonrInitCntr = 12 (AND Gate Fault)
      |     4 = 0000 0100 = Bit 2 = Fault Occured Between TmplMonrInitCntr = 14 ~ 15
      |     8 = 0000 1000 = Bit 3 = Fault Occured at TmplMonrInitCntr            = 17  (POE Fault)
      |   16 = 0001 0000 = Bit 4 = Fault Occured at TmplMonrInitCntr            = 18 (WD_STATE Fault)
      |   32 = 0010 0000 = Bit 5 = Fault Occured at TmplMonrInitCntr            = 20 (Edge/Valid Write Fault)
      |   64 = 0100 0000 = Bit 6 = Fault Occured at TmplMonrInitCntr            = 52 (POE + Non-WD Fault)
      | 128 = 1000 0000 = Bit 7 = Fault Occured at TmplMonrInitCntr            = 52 (POE + WD Fault)
  Action Port : ActionPort  ActionType=then
  Bitwise Operator2 : simulink/Logic and Bit Operations/Bitwise Operator  logicop=OR  UseBitMask=off  NumInputPorts=2  BitMask=bin2dec('00001111')  BitMaskRealWorld=Stored Integer
  CopyRight1 : Subsystem  Description=|  mask(Copyright Information){none=on}
      | Copyright info block.                                               
      |                                                                     
      | Place copyright information at the top of every subsystem in design.
      mask prompts: none "No parameters"
      mask help: Place copyright information at the top of every subsystem in design.
      mask Display:
      | NxtrConf = 'Nexteer Confidential';
      | 
      | sys = bdroot; %handle for the current model ("system")
      | first = get_param(sys,'Created');
      | first = first(end-3:end);  %year is last four digits
      | 
      | last = get_param(sys,'LastModifiedDate');
      | if isempty(last)
      |     last = datestr(now,'yyyy');
      | else
      |     last = last(end-3:end);
      | end
      | 
      | if strcmp(first,last)
      |     fprintf('%s -- Copyright %s Nexteer',NxtrConf,first)
      | else
      |     fprintf('%s -- %s%s- %s Nexteer',NxtrConf,char(169),first,last)
      | end
  Data Store Read3 : DataStoreRead  DataStoreName=TmplMonrNtc40PrmByte  DataStoreElements=TmplMonrNtc40PrmByte
  Data Store Write1 : DataStoreWrite  DataStoreName=TmplMonrNtc40PrmByte
  NtcStInfo : Constant  Value=32  OutDataTypeStr=uint8
  wires:
  Bitwise Operator2/1 -> Data Store Write1/1
  Data Store Read3/1 -> Bitwise Operator2/1
  NtcStInfo/1 -> Bitwise Operator2/2

== system ES005A_TmplMonr/TmplMonr/TmplMonrPer1/TMF Init Test/20/Spi_ReadIB ==
  note: Read Buffer - Simulation Purpose Only
      |
      |
      |
      |                            00001011
  Channel : Inport
  Constant1 : Constant  Value=11  OutDataTypeStr=uint16
  CopyRight1 : Subsystem  Description=|  mask(Copyright Information){none=on}
      | Copyright info block.                                               
      |                                                                     
      | Place copyright information at the top of every subsystem in design.
      mask prompts: none "No parameters"
      mask help: Place copyright information at the top of every subsystem in design.
      mask Display:
      | NxtrConf = 'Nexteer Confidential';
      | 
      | sys = bdroot; %handle for the current model ("system")
      | first = get_param(sys,'Created');
      | first = first(end-3:end);  %year is last four digits
      | 
      | last = get_param(sys,'LastModifiedDate');
      | if isempty(last)
      |     last = datestr(now,'yyyy');
      | else
      |     last = last(end-3:end);
      | end
      | 
      | if strcmp(first,last)
      |     fprintf('%s -- Copyright %s Nexteer',NxtrConf,first)
      | else
      |     fprintf('%s -- %s%s- %s Nexteer',NxtrConf,char(169),first,last)
      | end
  Terminator : Terminator
  Rx : Outport
  wires:
  Constant1/1 -> Rx/1
  Channel/1 -> Terminator/1

== system ES005A_TmplMonr/TmplMonr/TmplMonrPer1/TMF Init Test/21-51/CopyRight1 ==

== system ES005A_TmplMonr/TmplMonr/TmplMonrPer1/TMF Init Test/52/CopyRight1 ==

== system ES005A_TmplMonr/TmplMonr/TmplMonrPer1/TMF Init Test/52/Fault Condition - WD Run Fault ==
  Action Port : ActionPort  ActionType=else
  CopyRight1 : Subsystem  Description=|  mask(Copyright Information){none=on}
      | Copyright info block.                                               
      |                                                                     
      | Place copyright information at the top of every subsystem in design.
      mask prompts: none "No parameters"
      mask help: Place copyright information at the top of every subsystem in design.
      mask Display:
      | NxtrConf = 'Nexteer Confidential';
      | 
      | sys = bdroot; %handle for the current model ("system")
      | first = get_param(sys,'Created');
      | first = first(end-3:end);  %year is last four digits
      | 
      | last = get_param(sys,'LastModifiedDate');
      | if isempty(last)
      |     last = datestr(now,'yyyy');
      | else
      |     last = last(end-3:end);
      | end
      | 
      | if strcmp(first,last)
      |     fprintf('%s -- Copyright %s Nexteer',NxtrConf,first)
      | else
      |     fprintf('%s -- %s%s- %s Nexteer',NxtrConf,char(169),first,last)
      | end
  Data Store Read1 : DataStoreRead  DataStoreName=TmplMonrSpiReadWrOrderFlg1
  If : If  IfExpression=u1 == 0
  Merge1 : Merge
  Merge2 : Merge
  "TmplMonrSpiReadWrOrderFlg1 = 0 (Read Cmd) " : Subsystem
  TmplMonrSpiReadWrOrderFlg1 = 1 (Read Buffer) : Subsystem
  TmplMonrInitCntr : Outport
  TmplMonrIninTestCmpl : Outport  Port=2
  wires:
  If/1 -> "TmplMonrSpiReadWrOrderFlg1 = 0 (Read Cmd) "/Action
  If/2 -> TmplMonrSpiReadWrOrderFlg1 = 1 (Read Buffer)/Action
  Data Store Read1/1 -> If/1
  Merge1/1 -> TmplMonrInitCntr/1
  "TmplMonrSpiReadWrOrderFlg1 = 0 (Read Cmd) "/1(TmplMonrIninCntr) -> Merge1/1
  TmplMonrSpiReadWrOrderFlg1 = 1 (Read Buffer)/1(TmplMonrIninCntr) -> Merge1/2
  "TmplMonrSpiReadWrOrderFlg1 = 0 (Read Cmd) "/2(TmplMonrIninTestCmpl) -> Merge2/1
  TmplMonrSpiReadWrOrderFlg1 = 1 (Read Buffer)/2(TmplMonrIninTestCmpl) -> Merge2/2
  Merge2/1 -> TmplMonrIninTestCmpl/1

== system ES005A_TmplMonr/TmplMonr/TmplMonrPer1/TMF Init Test/52/IoHwAb_GetGpioPwrOutpEnaFb ==
  CopyRight1 : Subsystem  Description=|  mask(Copyright Information){none=on}
      | Copyright info block.                                               
      |                                                                     
      | Place copyright information at the top of every subsystem in design.
      mask prompts: none "No parameters"
      mask help: Place copyright information at the top of every subsystem in design.
      mask Display:
      | NxtrConf = 'Nexteer Confidential';
      | 
      | sys = bdroot; %handle for the current model ("system")
      | first = get_param(sys,'Created');
      | first = first(end-3:end);  %year is last four digits
      | 
      | last = get_param(sys,'LastModifiedDate');
      | if isempty(last)
      |     last = datestr(now,'yyyy');
      | else
      |     last = last(end-3:end);
      | end
      | 
      | if strcmp(first,last)
      |     fprintf('%s -- Copyright %s Nexteer',NxtrConf,first)
      | else
      |     fprintf('%s -- %s%s- %s Nexteer',NxtrConf,char(169),first,last)
      | end
  Ground : Ground
  PinSt : Outport
  wires:
  Ground/1 -> PinSt/1

== system ES005A_TmplMonr/TmplMonr/TmplMonrPer1/TMF Init Test/52/Normal Condition ==
  Action Port : ActionPort  ActionType=then
  Constant1 : Constant  OutDataTypeStr=boolean
  Constant2 : Constant  OutDataTypeStr=uint8
  Constant3 : Constant  Value=0  OutDataTypeStr=boolean
  Constant4 : Constant  OutDataTypeStr=boolean
  CopyRight1 : Subsystem  Description=|  mask(Copyright Information){none=on}
      | Copyright info block.                                               
      |                                                                     
      | Place copyright information at the top of every subsystem in design.
      mask prompts: none "No parameters"
      mask help: Place copyright information at the top of every subsystem in design.
      mask Display:
      | NxtrConf = 'Nexteer Confidential';
      | 
      | sys = bdroot; %handle for the current model ("system")
      | first = get_param(sys,'Created');
      | first = first(end-3:end);  %year is last four digits
      | 
      | last = get_param(sys,'LastModifiedDate');
      | if isempty(last)
      |     last = datestr(now,'yyyy');
      | else
      |     last = last(end-3:end);
      | end
      | 
      | if strcmp(first,last)
      |     fprintf('%s -- Copyright %s Nexteer',NxtrConf,first)
      | else
      |     fprintf('%s -- %s%s- %s Nexteer',NxtrConf,char(169),first,last)
      | end
  Data Store Write : DataStoreWrite  DataStoreName=TmplMonrSpiReadWrOrderFlg1
  Data Store Write2 : DataStoreWrite  DataStoreName=TmplMonrIninTestCmplFlg
      settings: AttributesFormatString=%<Name>
  TmplMonrIninCntr : Outport
  TmplMonrIninTestCmpl : Outport  Port=2
  wires:
  Constant2/1 -> TmplMonrIninCntr/1
  Constant1/1 -> TmplMonrIninTestCmpl/1
  Constant3/1 -> Data Store Write/1
  Constant4/1 -> Data Store Write2/1

== system ES005A_TmplMonr/TmplMonr/TmplMonrPer1/TMF Init Test/52/Set NTC 0x040 Note: Run last ==
  note: NTCNR_0X040
      | Parameters:
      |     1 = 0000 0001 = Bit 0 = Fault Occured Between TmplMonrInitCntr =  9 ~ 10
      |     2 = 0000 0010 = Bit 1 = Fault Occured Between TmplMonrInitCntr = 12 (AND Gate Fault)
      |     4 = 0000 0100 = Bit 2 = Fault Occured Between TmplMonrInitCntr = 14 ~ 15
      |     8 = 0000 1000 = Bit 3 = Fault Occured at TmplMonrInitCntr            = 17  (POE Fault)
      |   16 = 0001 0000 = Bit 4 = Fault Occured at TmplMonrInitCntr            = 18 (WD_STATE Fault)
      |   32 = 0010 0000 = Bit 5 = Fault Occured at TmplMonrInitCntr            = 20 (Edge/Valid Write Fault)
      |   64 = 0100 0000 = Bit 6 = Fault Occured at TmplMonrInitCntr            = 52 (POE + Non-WD Fault)
      | 128 = 1000 0000 = Bit 7 = Fault Occured at TmplMonrInitCntr            = 52 (POE + WD Fault)
  Data Store Read2 : DataStoreRead  DataStoreName=TmplMonrNtc40PrmByte  DataStoreElements=TmplMonrNtc40PrmByte
  FAILED = 1 : Subsystem
  If : If  IfExpression=u1 == 0
  PASSED = 0 : Subsystem
  wires:
  Data Store Read2/1 -> If/1, FAILED = 1/1(NtcStInfo)
  If/1 -> PASSED = 0/Action
  If/2 -> FAILED = 1/Action

== system ES005A_TmplMonr/TmplMonr/TmplMonrPer1/TMF Init Test/9-10, 14-16/CopyRight1 ==

== system ES005A_TmplMonr/TmplMonr/TmplMonrPer1/TMF Init Test/9-10, 14-16/IoHwAb_GetGpioPwrOutpEnaFb1 ==
  Action Port : ActionPort  ActionType=then
  CopyRight1 : Subsystem  Description=|  mask(Copyright Information){none=on}
      | Copyright info block.                                               
      |                                                                     
      | Place copyright information at the top of every subsystem in design.
      mask prompts: none "No parameters"
      mask help: Place copyright information at the top of every subsystem in design.
      mask Display:
      | NxtrConf = 'Nexteer Confidential';
      | 
      | sys = bdroot; %handle for the current model ("system")
      | first = get_param(sys,'Created');
      | first = first(end-3:end);  %year is last four digits
      | 
      | last = get_param(sys,'LastModifiedDate');
      | if isempty(last)
      |     last = datestr(now,'yyyy');
      | else
      |     last = last(end-3:end);
      | end
      | 
      | if strcmp(first,last)
      |     fprintf('%s -- Copyright %s Nexteer',NxtrConf,first)
      | else
      |     fprintf('%s -- %s%s- %s Nexteer',NxtrConf,char(169),first,last)
      | end
  Fault Condition - WD Signal : Subsystem  RequirementInfo={'linktype_rmi_doors' '0000c46a (/ESG Group/FDD Module Requirements/EA4 Specific/ES005A_TmplMonr)' '#ES005A_158' 'true' 'REQ: ES005A_158' '' ; 'linktype_rmi_doors' '0000c46a (/ESG Group/FDD Module Requirements/EA4 Specific/ES005A_TmplMonr)' '#ES005A_163' 'true' 'REQ: ES005A_163' '' ; 'linktype_rmi_doors' '0000c46a (/ESG Group/FDD Module Requirements/EA4 Specific/ES005A_TmplMonr)' '#ES005A_172' 'true' 'REQ: ES005A_172' '' } %GIDa_89a4d9ae_99ea_4011_b803_c994c7645272
  If1 : If  RequirementInfo={'linktype_rmi_doors' '0000c46a (/ESG Group/FDD Module Requirements/EA4 Specific/ES005A_TmplMonr)' '#ES005A_163' 'true' 'REQ: ES005A_163' '' ; 'linktype_rmi_doors' '0000c46a (/ESG Group/FDD Module Requirements/EA4 Specific/ES005A_TmplMonr)' '#ES005A_172' 'true' 'REQ: ES005A_172' '' } %GIDa_4f483320_e134_42eb_ab01_bf1264f50d52  IfExpression=u1 ~= 1  ShowElse=off
  IoHwAb_GetGpioPwrOutpEnaFb : Subsystem
  wires:
  If1/1 -> Fault Condition - WD Signal/Action
  IoHwAb_GetGpioPwrOutpEnaFb/1(PinSt) -> If1/1

== system ES005A_TmplMonr/TmplMonr/TmplMonrPer1/TMF Init Test/Default/CopyRight1 ==

== system ES005A_TmplMonr/TmplMonr/TmplMonrPer1/TMF Init Test/IoHwAb_SetGpioTmplMonrWdg/CopyRight1 ==

== system ES005A_TmplMonr/TmplMonr/TmplMonrPer1/TMF Init Test/IoHwAb_SetGpioTmplMonrWdg/IoHwAb_SetGpioTmplMonrWdg ==
  PinSt : Inport
  CopyRight1 : Subsystem  Description=|  mask(Copyright Information){none=on}
      | Copyright info block.                                               
      |                                                                     
      | Place copyright information at the top of every subsystem in design.
      mask prompts: none "No parameters"
      mask help: Place copyright information at the top of every subsystem in design.
      mask Display:
      | NxtrConf = 'Nexteer Confidential';
      | 
      | sys = bdroot; %handle for the current model ("system")
      | first = get_param(sys,'Created');
      | first = first(end-3:end);  %year is last four digits
      | 
      | last = get_param(sys,'LastModifiedDate');
      | if isempty(last)
      |     last = datestr(now,'yyyy');
      | else
      |     last = last(end-3:end);
      | end
      | 
      | if strcmp(first,last)
      |     fprintf('%s -- Copyright %s Nexteer',NxtrConf,first)
      | else
      |     fprintf('%s -- %s%s- %s Nexteer',NxtrConf,char(169),first,last)
      | end
  Terminator : Terminator
  wires:
  PinSt/1 -> Terminator/1

== system ES005A_TmplMonr/TmplMonr/TmplMonrPer1/TMF Init Test/nError Signal Control/CopyRight1 ==
